simulink model "t05_balancing"  (R2024b)
settings: Solver=ode23t  StartTime=0.0  StopTime=6  RelTol=1e-3  AbsTol=1e-3  EnableMultiTasking=on
InitFcn:
  | run('Parameters_pntcld.m');
model workspace (MAT data in the model file):
  A = 0.4
  Critical_Velocity = 0.01
  Damping_Factor = 1000
  Dynamic_Friction = 0.5
  Heigth_brick : Simulink.Parameter (value not decoded)
  Heigth_ramp : Simulink.Parameter (value not decoded)
  Length_brick : Simulink.Parameter (value not decoded)
  Length_ramp : Simulink.Parameter (value not decoded)
  Length_torso : Simulink.Parameter (value not decoded)
  Lower_limbs : Simulink.Parameter (value not decoded)
  Static_Friction = 0.7
  Stiffnesscoefficient = 10000
  Transition_Region_Width = 0.02
  Upper_limbs : Simulink.Parameter (value not decoded)
  Width_brick : Simulink.Parameter (value not decoded)
  Width_ramp : Simulink.Parameter (value not decoded)
  Width_torso : Simulink.Parameter (value not decoded)
  f = 1.5
  max_Joint_change = 100
  r_foot : Simulink.Parameter (value not decoded)
  sampleTime : Simulink.Parameter (value not decoded)
  t_leg : Simulink.Parameter (value not decoded)
  theta : Simulink.Parameter (value not decoded)
  transferFunVal : Simulink.Parameter (value not decoded)
symbols that are objects in the model workspace (value not decoded): Length_torso, Lower_limbs, t_leg, transferFunVal, Upper_limbs, Width_torso
undefined symbols (not defined in the file): X, Y, Z
libraries: sm_lib x87, nesl_utility x17
(part 3 of 3)

== system t05_balancing/Front Left Leg/Upper Limb ==
  BaseUpperLimb : sm_lib/Body Elements/Brick Solid  BrickDimensions=[t_leg t_leg L]  BrickDimensionsUnits=m  ExportEntireGeometry=off  InertiaType=CalculateFromGeometry  BasedOnType=Density  Density=1000  DensityUnits=kg/m^3  Mass=1  MassUnits=kg  CenterOfMass=[0 0 0]  CenterOfMassUnits=m  MomentsOfInertia=[1 1 1]  MomentsOfInertiaUnits=kg*m^2  ProductsOfInertia=[0 0 0]  ProductsOfInertiaUnits=kg*m^2  GraphicType=FromGeometry  MarkerShape=Sphere  MarkerSize=10  GraphicVisPropType=SimpleVisualProperties  GraphicDiffuseColor=[0.502 0.502 0.502]  GraphicOpacity=1  GraphicSpecularColor=[0.5 0.5 0.5 1.0]  GraphicAmbientColor=[0.15 0.15 0.15 1.0]  GraphicEmissiveColor=[0.0 0.0 0.0 1.0]  GraphicShininess=75  DoExposeReferenceFrame=off  SerializedFrames=<Frames><Frame><Id>Frame1</Id><Value><Name>B</Name><Origin><Source>GeometricFeature</Source><FeatureName>+z surface</FeatureName></Origin><PrimaryAxis><DefinedDirection>+Z</DefinedDirection><Source>ReferenceFrame</Source><SourceDirection>+Z</SourceDirection><FeatureName></FeatureName></PrimaryAxis><SecondaryAxis><DefinedDirection>+X</DefinedDirection><Source>ReferenceFrame</Source><SourceDirection>+X</SourceDirection><FeatureName></FeatureName></SecondaryAxis></Value></Frame><Frame><Id>Frame2</Id><Value><Name>F</Name><Origin><Source>GeometricFeature</Source><FeatureName>-z surface</FeatureName></Origin><PrimaryAxis><DefinedDirection>+Z</DefinedDirection><Source>ReferenceFrame</Source><SourceDirection>+Z</SourceDirection><FeatureName></FeatureName></PrimaryAxis><SecondaryAxis><DefinedDirection>+X</DefinedDirection><Source>ReferenceFrame</Source><SourceDirection>+X</SourceDirection><FeatureName></FeatureName></SecondaryAxis></Value></Frame></Frames>
  Transform Shoulder : sm_lib/Frames and Transforms/Rigid Transform  RotationMethod=StandardAxis  FollAlignAxisA=+X  BaseAlignAxisA=+Y  FollAlignAxisB=+Y  BaseAlignAxisB=+Z  RotationStandardAxis=+X  RotationAngle=-90  RotationAngleUnits=deg  RotationArbitraryAxis=[0 0 1]  RotationSequenceAxes=FollowerAxes  RotationSequence=XYX  RotationSequenceAngles=[0 0 0]  RotationSequenceAnglesUnits=deg  RotationMatrix=[1 0 0;0 1 0;0 0 1]  Quaternion=[1 0 0 0]  TranslationMethod=StandardAxis  TranslationCartesianOffset=[0 0 0]  TranslationCartesianOffsetUnits=m  TranslationStandardAxis=+Z  TranslationStandardOffset=0  TranslationStandardOffsetUnits=m  TranslationROffset=0  TranslationROffsetUnits=m  TranslationThetaOffset=0  TranslationThetaOffsetUnits=deg  TranslationZOffset=0  TranslationZOffsetUnits=m
  Transform Upper Knee : sm_lib/Frames and Transforms/Rigid Transform  RotationMethod=StandardAxis  FollAlignAxisA=+X  BaseAlignAxisA=+Y  FollAlignAxisB=+Y  BaseAlignAxisB=+Z  RotationStandardAxis=+X  RotationAngle=-90  RotationAngleUnits=deg  RotationArbitraryAxis=[0 0 1]  RotationSequenceAxes=FollowerAxes  RotationSequence=XYX  RotationSequenceAngles=[0 0 0]  RotationSequenceAnglesUnits=deg  RotationMatrix=[1 0 0;0 1 0;0 0 1]  Quaternion=[1 0 0 0]  TranslationMethod=StandardAxis  TranslationCartesianOffset=[0 0 0]  TranslationCartesianOffsetUnits=m  TranslationStandardAxis=+Z  TranslationStandardOffset=0  TranslationStandardOffsetUnits=m  TranslationROffset=0  TranslationROffsetUnits=m  TranslationThetaOffset=0  TranslationThetaOffsetUnits=deg  TranslationZOffset=0  TranslationZOffsetUnits=m
  U : PMIOPort  Side=Left
  L : PMIOPort  Port=2  Side=Right
  connections:
  L/RConn1 -- Transform Upper Knee/RConn1
  U/RConn1 -- Transform Shoulder/RConn1
  BaseUpperLimb/LConn1 -- Transform Shoulder/LConn1
  BaseUpperLimb/RConn1 -- Transform Upper Knee/LConn1

== system t05_balancing/Front Right Leg/Lower Limb ==
  BaseLowerLimb : sm_lib/Body Elements/Brick Solid  BrickDimensions=[t_leg t_leg L]  BrickDimensionsUnits=m  ExportEntireGeometry=off  InertiaType=CalculateFromGeometry  BasedOnType=Density  Density=1000  DensityUnits=kg/m^3  Mass=1  MassUnits=kg  CenterOfMass=[0 0 0]  CenterOfMassUnits=m  MomentsOfInertia=[1 1 1]  MomentsOfInertiaUnits=kg*m^2  ProductsOfInertia=[0 0 0]  ProductsOfInertiaUnits=kg*m^2  GraphicType=FromGeometry  MarkerShape=Sphere  MarkerSize=10  GraphicVisPropType=SimpleVisualProperties  GraphicDiffuseColor=[0.5 0.5 0.5]  GraphicOpacity=1  GraphicSpecularColor=[0.5 0.5 0.5 1.0]  GraphicAmbientColor=[0.15 0.15 0.15 1.0]  GraphicEmissiveColor=[0.0 0.0 0.0 1.0]  GraphicShininess=75  DoExposeReferenceFrame=off  SerializedFrames=<Frames><Frame><Id>Frame1</Id><Value><Name>B</Name><Origin><Source>GeometricFeature</Source><FeatureName>+z surface</FeatureName></Origin><PrimaryAxis><DefinedDirection>+Z</DefinedDirection><Source>ReferenceFrame</Source><SourceDirection>+Z</SourceDirection><FeatureName></FeatureName></PrimaryAxis><SecondaryAxis><DefinedDirection>+X</DefinedDirection><Source>ReferenceFrame</Source><SourceDirection>+X</SourceDirection><FeatureName></FeatureName></SecondaryAxis></Value></Frame><Frame><Id>Frame2</Id><Value><Name>F</Name><Origin><Source>GeometricFeature</Source><FeatureName>-z surface</FeatureName></Origin><PrimaryAxis><DefinedDirection>+Z</DefinedDirection><Source>ReferenceFrame</Source><SourceDirection>+Z</SourceDirection><FeatureName></FeatureName></PrimaryAxis><SecondaryAxis><DefinedDirection>+X</DefinedDirection><Source>ReferenceFrame</Source><SourceDirection>+X</SourceDirection><FeatureName></FeatureName></SecondaryAxis></Value></Frame></Frames>
  Transform Shoulder : sm_lib/Frames and Transforms/Rigid Transform  RotationMethod=StandardAxis  FollAlignAxisA=+X  BaseAlignAxisA=+Y  FollAlignAxisB=+Y  BaseAlignAxisB=+Z  RotationStandardAxis=+X  RotationAngle=-90  RotationAngleUnits=deg  RotationArbitraryAxis=[0 0 1]  RotationSequenceAxes=FollowerAxes  RotationSequence=XYX  RotationSequenceAngles=[0 0 0]  RotationSequenceAnglesUnits=deg  RotationMatrix=[1 0 0;0 1 0;0 0 1]  Quaternion=[1 0 0 0]  TranslationMethod=StandardAxis  TranslationCartesianOffset=[0 0 0]  TranslationCartesianOffsetUnits=m  TranslationStandardAxis=+Z  TranslationStandardOffset=0  TranslationStandardOffsetUnits=m  TranslationROffset=0  TranslationROffsetUnits=m  TranslationThetaOffset=0  TranslationThetaOffsetUnits=deg  TranslationZOffset=0  TranslationZOffsetUnits=m
  Transform Upper Knee : sm_lib/Frames and Transforms/Rigid Transform  RotationMethod=StandardAxis  FollAlignAxisA=+X  BaseAlignAxisA=+Y  FollAlignAxisB=+Y  BaseAlignAxisB=+Z  RotationStandardAxis=+X  RotationAngle=-90  RotationAngleUnits=deg  RotationArbitraryAxis=[0 0 1]  RotationSequenceAxes=FollowerAxes  RotationSequence=XYX  RotationSequenceAngles=[0 0 0]  RotationSequenceAnglesUnits=deg  RotationMatrix=[1 0 0;0 1 0;0 0 1]  Quaternion=[1 0 0 0]  TranslationMethod=StandardAxis  TranslationCartesianOffset=[0 0 0]  TranslationCartesianOffsetUnits=m  TranslationStandardAxis=+Z  TranslationStandardOffset=0  TranslationStandardOffsetUnits=m  TranslationROffset=0  TranslationROffsetUnits=m  TranslationThetaOffset=0  TranslationThetaOffsetUnits=deg  TranslationZOffset=0  TranslationZOffsetUnits=m
  U : PMIOPort  Side=Left
  L : PMIOPort  Port=2  Side=Right
  connections:
  BaseLowerLimb/LConn1 -- Transform Shoulder/LConn1
  Transform Shoulder/RConn1 -- U/RConn1
  L/RConn1 -- Transform Upper Knee/RConn1
  BaseLowerLimb/RConn1 -- Transform Upper Knee/LConn1

== system t05_balancing/Front Right Leg/Upper Limb ==
  BaseUpperLimb : sm_lib/Body Elements/Brick Solid  BrickDimensions=[t_leg t_leg L]  BrickDimensionsUnits=m  ExportEntireGeometry=off  InertiaType=CalculateFromGeometry  BasedOnType=Density  Density=1000  DensityUnits=kg/m^3  Mass=1  MassUnits=kg  CenterOfMass=[0 0 0]  CenterOfMassUnits=m  MomentsOfInertia=[1 1 1]  MomentsOfInertiaUnits=kg*m^2  ProductsOfInertia=[0 0 0]  ProductsOfInertiaUnits=kg*m^2  GraphicType=FromGeometry  MarkerShape=Sphere  MarkerSize=10  GraphicVisPropType=SimpleVisualProperties  GraphicDiffuseColor=[0.502 0.502 0.502]  GraphicOpacity=1  GraphicSpecularColor=[0.5 0.5 0.5 1.0]  GraphicAmbientColor=[0.15 0.15 0.15 1.0]  GraphicEmissiveColor=[0.0 0.0 0.0 1.0]  GraphicShininess=75  DoExposeReferenceFrame=off  SerializedFrames=<Frames><Frame><Id>Frame1</Id><Value><Name>B</Name><Origin><Source>GeometricFeature</Source><FeatureName>+z surface</FeatureName></Origin><PrimaryAxis><DefinedDirection>+Z</DefinedDirection><Source>ReferenceFrame</Source><SourceDirection>+Z</SourceDirection><FeatureName></FeatureName></PrimaryAxis><SecondaryAxis><DefinedDirection>+X</DefinedDirection><Source>ReferenceFrame</Source><SourceDirection>+X</SourceDirection><FeatureName></FeatureName></SecondaryAxis></Value></Frame><Frame><Id>Frame2</Id><Value><Name>F</Name><Origin><Source>GeometricFeature</Source><FeatureName>-z surface</FeatureName></Origin><PrimaryAxis><DefinedDirection>+Z</DefinedDirection><Source>ReferenceFrame</Source><SourceDirection>+Z</SourceDirection><FeatureName></FeatureName></PrimaryAxis><SecondaryAxis><DefinedDirection>+X</DefinedDirection><Source>ReferenceFrame</Source><SourceDirection>+X</SourceDirection><FeatureName></FeatureName></SecondaryAxis></Value></Frame></Frames>
  Transform Shoulder : sm_lib/Frames and Transforms/Rigid Transform  RotationMethod=StandardAxis  FollAlignAxisA=+X  BaseAlignAxisA=+Y  FollAlignAxisB=+Y  BaseAlignAxisB=+Z  RotationStandardAxis=+X  RotationAngle=-90  RotationAngleUnits=deg  RotationArbitraryAxis=[0 0 1]  RotationSequenceAxes=FollowerAxes  RotationSequence=XYX  RotationSequenceAngles=[0 0 0]  RotationSequenceAnglesUnits=deg  RotationMatrix=[1 0 0;0 1 0;0 0 1]  Quaternion=[1 0 0 0]  TranslationMethod=StandardAxis  TranslationCartesianOffset=[0 0 0]  TranslationCartesianOffsetUnits=m  TranslationStandardAxis=+Z  TranslationStandardOffset=0  TranslationStandardOffsetUnits=m  TranslationROffset=0  TranslationROffsetUnits=m  TranslationThetaOffset=0  TranslationThetaOffsetUnits=deg  TranslationZOffset=0  TranslationZOffsetUnits=m
  Transform Upper Knee : sm_lib/Frames and Transforms/Rigid Transform  RotationMethod=StandardAxis  FollAlignAxisA=+X  BaseAlignAxisA=+Y  FollAlignAxisB=+Y  BaseAlignAxisB=+Z  RotationStandardAxis=+X  RotationAngle=-90  RotationAngleUnits=deg  RotationArbitraryAxis=[0 0 1]  RotationSequenceAxes=FollowerAxes  RotationSequence=XYX  RotationSequenceAngles=[0 0 0]  RotationSequenceAnglesUnits=deg  RotationMatrix=[1 0 0;0 1 0;0 0 1]  Quaternion=[1 0 0 0]  TranslationMethod=StandardAxis  TranslationCartesianOffset=[0 0 0]  TranslationCartesianOffsetUnits=m  TranslationStandardAxis=+Z  TranslationStandardOffset=0  TranslationStandardOffsetUnits=m  TranslationROffset=0  TranslationROffsetUnits=m  TranslationThetaOffset=0  TranslationThetaOffsetUnits=deg  TranslationZOffset=0  TranslationZOffsetUnits=m
  U : PMIOPort  Side=Left
  L : PMIOPort  Port=2  Side=Right
  connections:
  L/RConn1 -- Transform Upper Knee/RConn1
  U/RConn1 -- Transform Shoulder/RConn1
  BaseUpperLimb/LConn1 -- Transform Shoulder/LConn1
  BaseUpperLimb/RConn1 -- Transform Upper Knee/LConn1

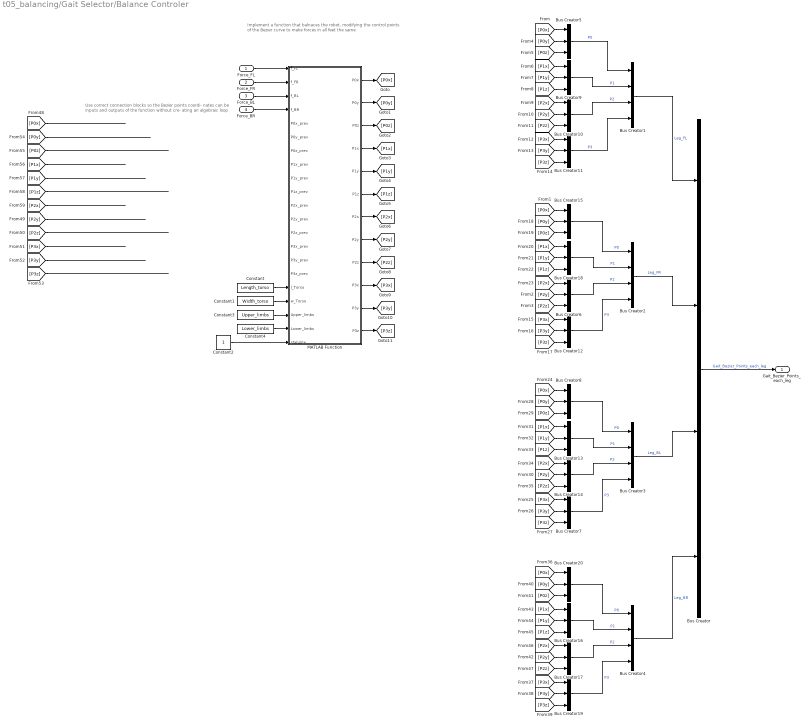
== system t05_balancing/Gait Selector/Balance Controler ==
  note: Implement a function that balnaces the robot, modifying
      | the control points of the Bezier curve to make forces in all
      | feet the same
  note: Use correct connection blocks so the Bezier points coordi-
      | nates can be inputs and outputs of the function without cre-
      | ating an algebraic loop
  Force_FL : Inport
  Force_FR : Inport  Port=2
  Force_BL : Inport  Port=3
  Force_BR : Inport  Port=4
  Bus Creator{,1..4} (5 alike) : BusCreator  Inputs=4
  Bus Creator{5..20} (16 alike) : BusCreator  Inputs=3
  Constant : Constant  Value=Length_torso
  Constant1 : Constant  Value=Width_torso
  Constant2 : Constant
  Constant3 : Constant  Value=Upper_limbs
  Constant4 : Constant  Value=Lower_limbs
  MATLAB Function : MATLAB Function  TreatAsAtomicUnit=on
  Gait_Bezier_Points_each_leg : Outport
  wires:
  Constant2/1 -> MATLAB Function/21(stabilize)
  Constant4/1 -> MATLAB Function/20(Lower_limbs)
  Constant3/1 -> MATLAB Function/19(Upper_limbs)
  ? -> MATLAB Function/13(P2z_prev)
  ? -> MATLAB Function/14(P3x_prev)
  ? -> MATLAB Function/10(P1z_prev)
  ? -> MATLAB Function/8(P1x_prev)
  ? -> MATLAB Function/12(P2y_prev)
  ? -> MATLAB Function/9(P1y_prev)
  ? -> MATLAB Function/11(P2x_prev)
  ? -> MATLAB Function/5(P0x_prev)
  ? -> MATLAB Function/15(P3y_prev)
  ? -> MATLAB Function/7(P0z_prev)
  ? -> MATLAB Function/16(P3z_prev)
  ? -> MATLAB Function/6(P0y_prev)
  [P3y] -> ?
  [P3z] -> ?
  [P3x] -> ?
  [P2x] -> ?
  [P2z] -> ?
  [P2y] -> ?
  Bus Creator20/1 -> Bus Creator4/1  "P0"
  Bus Creator16/1 -> Bus Creator4/2  "P1"
  Bus Creator17/1 -> Bus Creator4/3  "P2"
  Bus Creator19/1 -> Bus Creator4/4  "P3"
  [P0x] -> Bus Creator20/1
  [P0y] -> Bus Creator20/2
  [P0z] -> Bus Creator20/3
  [P1y] -> Bus Creator16/2
  [P1x] -> Bus Creator16/1
  [P1z] -> Bus Creator16/3
  [P3z] -> Bus Creator19/3
  [P3x] -> Bus Creator19/1
  [P3y] -> Bus Creator19/2
  [P2z] -> Bus Creator17/3
  [P2y] -> Bus Creator17/2
  [P2x] -> Bus Creator17/1
  [P2x] -> Bus Creator14/1
  [P2y] -> Bus Creator14/2
  [P2z] -> Bus Creator14/3
  [P3y] -> Bus Creator7/2
  [P3x] -> Bus Creator7/1
  [P3z] -> Bus Creator7/3
  [P1z] -> Bus Creator13/3
  [P1x] -> Bus Creator13/1
  [P1y] -> Bus Creator13/2
  [P0z] -> Bus Creator8/3
  [P0y] -> Bus Creator8/2
  [P0x] -> Bus Creator8/1
  Bus Creator7/1 -> Bus Creator3/4  "P3"
  Bus Creator14/1 -> Bus Creator3/3  "P2"
  Bus Creator13/1 -> Bus Creator3/2  "P1"
  Bus Creator8/1 -> Bus Creator3/1  "P0"
  Bus Creator15/1 -> Bus Creator2/1  "P0"
  Bus Creator18/1 -> Bus Creator2/2  "P1"
  Bus Creator6/1 -> Bus Creator2/3  "P2"
  Bus Creator12/1 -> Bus Creator2/4  "P3"
  [P0x] -> Bus Creator15/1
  [P0y] -> Bus Creator15/2
  [P0z] -> Bus Creator15/3
  [P1y] -> Bus Creator18/2
  [P1x] -> Bus Creator18/1
  [P1z] -> Bus Creator18/3
  [P3z] -> Bus Creator12/3
  [P3x] -> Bus Creator12/1
  [P3y] -> Bus Creator12/2
  [P2z] -> Bus Creator6/3
  [P2y] -> Bus Creator6/2
  [P2x] -> Bus Creator6/1
  [P2x] -> Bus Creator10/1
  [P2y] -> Bus Creator10/2
  [P2z] -> Bus Creator10/3
  [P3y] -> Bus Creator11/2
  [P3x] -> Bus Creator11/1
  [P3z] -> Bus Creator11/3
  [P1z] -> Bus Creator9/3
  [P1x] -> Bus Creator9/1
  [P1y] -> Bus Creator9/2
  MATLAB Function/7(P2x) -> [P2x]
  MATLAB Function/8(P2y) -> [P2y]
  MATLAB Function/9(P2z) -> [P2z]
  MATLAB Function/12(P3z) -> [P3z]
  MATLAB Function/11(P3y) -> [P3y]
  MATLAB Function/10(P3x) -> [P3x]
  MATLAB Function/4(P1x) -> [P1x]
  MATLAB Function/5(P1y) -> [P1y]
  MATLAB Function/6(P1z) -> [P1z]
  MATLAB Function/3(P0z) -> [P0z]
  MATLAB Function/2(P0y) -> [P0y]
  [P0z] -> Bus Creator5/3
  [P0y] -> Bus Creator5/2
  [P0x] -> Bus Creator5/1
  Constant1/1 -> MATLAB Function/18(w_Torso)
  Constant/1 -> MATLAB Function/17(l_Torso)
  [P1z] -> ?
  [P1x] -> ?
  [P1y] -> ?
  [P0y] -> ?
  [P0z] -> ?
  [P0x] -> ?
  Force_BR/1 -> MATLAB Function/4(f_BR)
  Force_BL/1 -> MATLAB Function/3(f_BL)
  Force_FR/1 -> MATLAB Function/2(f_FR)
  Force_FL/1 -> MATLAB Function/1(f_FL)
  MATLAB Function/1(P0x) -> [P0x]
  Bus Creator11/1 -> Bus Creator1/4  "P3"
  Bus Creator10/1 -> Bus Creator1/3  "P2"
  Bus Creator9/1 -> Bus Creator1/2  "P1"
  Bus Creator5/1 -> Bus Creator1/1  "P0"
  Bus Creator/1 -> Gait_Bezier_Points_each_leg/1  "Gait_Bezier_Points_each_leg"
  Bus Creator4/1 -> Bus Creator/4  "Leg_BR"
  Bus Creator3/1 -> Bus Creator/3  "Leg_BL"
  Bus Creator2/1 -> Bus Creator/2  "Leg_FR"
  Bus Creator1/1 -> Bus Creator/1  "Leg_FL"

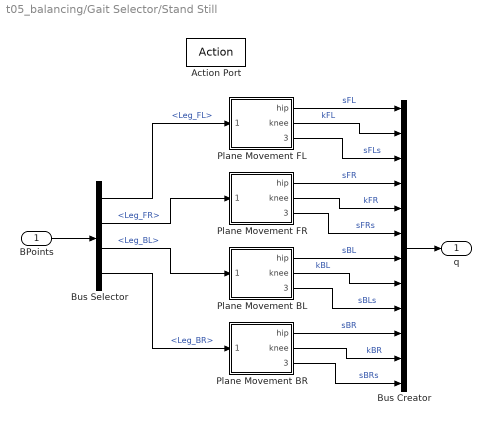
== system t05_balancing/Gait Selector/Stand Still ==
  BPoints : Inport
  Action Port : ActionPort  InitializeStates=reset  ActionPortLabel=case [ 0 ]:
  Bus Creator : BusCreator  Inputs=12
  Bus Selector : BusSelector  OutputSignals=Leg_FL,Leg_FR,Leg_BL,Leg_BR
  Plane Movement BL : Subsystem
  Plane Movement BR : Subsystem
  Plane Movement FL : Subsystem
  Plane Movement FR : Subsystem
  q : Outport
  wires:
  Bus Selector/4 -> Plane Movement BR/1(BPoints)  "<Leg_BR>"
  Bus Selector/3 -> Plane Movement BL/1(BPoints)  "<Leg_BL>"
  Bus Creator/1 -> q/1
  Plane Movement FL/1(hip) -> Bus Creator/1  "sFL"
  Plane Movement FR/1(hip) -> Bus Creator/4  "sFR"
  Plane Movement FL/2(knee) -> Bus Creator/2  "kFL"
  Plane Movement FR/2(knee) -> Bus Creator/5  "kFR"
  Plane Movement BL/2(knee) -> Bus Creator/8  "kBL"
  Plane Movement BL/1(hip) -> Bus Creator/7  "sBL"
  Plane Movement BR/2(knee) -> Bus Creator/11  "kBR"
  Plane Movement BR/1(hip) -> Bus Creator/10  "sBR"
  Plane Movement FL/3(HipLateral) -> Bus Creator/3  "sFLs"
  Plane Movement FR/3(HipLateral) -> Bus Creator/6  "sFRs"
  Plane Movement BL/3(HipLateral) -> Bus Creator/9  "sBLs"
  Plane Movement BR/3(HipLateral) -> Bus Creator/12  "sBRs"
  BPoints/1 -> Bus Selector/1
  Bus Selector/1 -> Plane Movement FL/1(BPoints)  "<Leg_FL>"
  Bus Selector/2 -> Plane Movement FR/1(BPoints)  "<Leg_FR>"

== system t05_balancing/Rear Left Leg/Lower Limb ==
  BaseLowerLimb : sm_lib/Body Elements/Brick Solid  BrickDimensions=[t_leg t_leg L]  BrickDimensionsUnits=m  ExportEntireGeometry=off  InertiaType=CalculateFromGeometry  BasedOnType=Density  Density=1000  DensityUnits=kg/m^3  Mass=1  MassUnits=kg  CenterOfMass=[0 0 0]  CenterOfMassUnits=m  MomentsOfInertia=[1 1 1]  MomentsOfInertiaUnits=kg*m^2  ProductsOfInertia=[0 0 0]  ProductsOfInertiaUnits=kg*m^2  GraphicType=FromGeometry  MarkerShape=Sphere  MarkerSize=10  GraphicVisPropType=SimpleVisualProperties  GraphicDiffuseColor=[0.5 0.5 0.5]  GraphicOpacity=1  GraphicSpecularColor=[0.5 0.5 0.5 1.0]  GraphicAmbientColor=[0.15 0.15 0.15 1.0]  GraphicEmissiveColor=[0.0 0.0 0.0 1.0]  GraphicShininess=75  DoExposeReferenceFrame=off  SerializedFrames=<Frames><Frame><Id>Frame1</Id><Value><Name>B</Name><Origin><Source>GeometricFeature</Source><FeatureName>+z surface</FeatureName></Origin><PrimaryAxis><DefinedDirection>+Z</DefinedDirection><Source>ReferenceFrame</Source><SourceDirection>+Z</SourceDirection><FeatureName></FeatureName></PrimaryAxis><SecondaryAxis><DefinedDirection>+X</DefinedDirection><Source>ReferenceFrame</Source><SourceDirection>+X</SourceDirection><FeatureName></FeatureName></SecondaryAxis></Value></Frame><Frame><Id>Frame2</Id><Value><Name>F</Name><Origin><Source>GeometricFeature</Source><FeatureName>-z surface</FeatureName></Origin><PrimaryAxis><DefinedDirection>+Z</DefinedDirection><Source>ReferenceFrame</Source><SourceDirection>+Z</SourceDirection><FeatureName></FeatureName></PrimaryAxis><SecondaryAxis><DefinedDirection>+X</DefinedDirection><Source>ReferenceFrame</Source><SourceDirection>+X</SourceDirection><FeatureName></FeatureName></SecondaryAxis></Value></Frame></Frames>
  Transform Shoulder : sm_lib/Frames and Transforms/Rigid Transform  RotationMethod=StandardAxis  FollAlignAxisA=+X  BaseAlignAxisA=+Y  FollAlignAxisB=+Y  BaseAlignAxisB=+Z  RotationStandardAxis=+X  RotationAngle=-90  RotationAngleUnits=deg  RotationArbitraryAxis=[0 0 1]  RotationSequenceAxes=FollowerAxes  RotationSequence=XYX  RotationSequenceAngles=[0 0 0]  RotationSequenceAnglesUnits=deg  RotationMatrix=[1 0 0;0 1 0;0 0 1]  Quaternion=[1 0 0 0]  TranslationMethod=StandardAxis  TranslationCartesianOffset=[0 0 0]  TranslationCartesianOffsetUnits=m  TranslationStandardAxis=+Z  TranslationStandardOffset=0  TranslationStandardOffsetUnits=m  TranslationROffset=0  TranslationROffsetUnits=m  TranslationThetaOffset=0  TranslationThetaOffsetUnits=deg  TranslationZOffset=0  TranslationZOffsetUnits=m
  Transform Upper Knee : sm_lib/Frames and Transforms/Rigid Transform  RotationMethod=StandardAxis  FollAlignAxisA=+X  BaseAlignAxisA=+Y  FollAlignAxisB=+Y  BaseAlignAxisB=+Z  RotationStandardAxis=+X  RotationAngle=-90  RotationAngleUnits=deg  RotationArbitraryAxis=[0 0 1]  RotationSequenceAxes=FollowerAxes  RotationSequence=XYX  RotationSequenceAngles=[0 0 0]  RotationSequenceAnglesUnits=deg  RotationMatrix=[1 0 0;0 1 0;0 0 1]  Quaternion=[1 0 0 0]  TranslationMethod=StandardAxis  TranslationCartesianOffset=[0 0 0]  TranslationCartesianOffsetUnits=m  TranslationStandardAxis=+Z  TranslationStandardOffset=0  TranslationStandardOffsetUnits=m  TranslationROffset=0  TranslationROffsetUnits=m  TranslationThetaOffset=0  TranslationThetaOffsetUnits=deg  TranslationZOffset=0  TranslationZOffsetUnits=m
  U : PMIOPort  Side=Left
  L : PMIOPort  Port=2  Side=Right
  connections:
  BaseLowerLimb/LConn1 -- Transform Shoulder/LConn1
  Transform Shoulder/RConn1 -- U/RConn1
  L/RConn1 -- Transform Upper Knee/RConn1
  BaseLowerLimb/RConn1 -- Transform Upper Knee/LConn1

== system t05_balancing/Rear Left Leg/Upper Limb ==
  BaseUpperLimb : sm_lib/Body Elements/Brick Solid  BrickDimensions=[t_leg t_leg L]  BrickDimensionsUnits=m  ExportEntireGeometry=off  InertiaType=CalculateFromGeometry  BasedOnType=Density  Density=1000  DensityUnits=kg/m^3  Mass=1  MassUnits=kg  CenterOfMass=[0 0 0]  CenterOfMassUnits=m  MomentsOfInertia=[1 1 1]  MomentsOfInertiaUnits=kg*m^2  ProductsOfInertia=[0 0 0]  ProductsOfInertiaUnits=kg*m^2  GraphicType=FromGeometry  MarkerShape=Sphere  MarkerSize=10  GraphicVisPropType=SimpleVisualProperties  GraphicDiffuseColor=[0.502 0.502 0.502]  GraphicOpacity=1  GraphicSpecularColor=[0.5 0.5 0.5 1.0]  GraphicAmbientColor=[0.15 0.15 0.15 1.0]  GraphicEmissiveColor=[0.0 0.0 0.0 1.0]  GraphicShininess=75  DoExposeReferenceFrame=off  SerializedFrames=<Frames><Frame><Id>Frame1</Id><Value><Name>B</Name><Origin><Source>GeometricFeature</Source><FeatureName>+z surface</FeatureName></Origin><PrimaryAxis><DefinedDirection>+Z</DefinedDirection><Source>ReferenceFrame</Source><SourceDirection>+Z</SourceDirection><FeatureName></FeatureName></PrimaryAxis><SecondaryAxis><DefinedDirection>+X</DefinedDirection><Source>ReferenceFrame</Source><SourceDirection>+X</SourceDirection><FeatureName></FeatureName></SecondaryAxis></Value></Frame><Frame><Id>Frame2</Id><Value><Name>F</Name><Origin><Source>GeometricFeature</Source><FeatureName>-z surface</FeatureName></Origin><PrimaryAxis><DefinedDirection>+Z</DefinedDirection><Source>ReferenceFrame</Source><SourceDirection>+Z</SourceDirection><FeatureName></FeatureName></PrimaryAxis><SecondaryAxis><DefinedDirection>+X</DefinedDirection><Source>ReferenceFrame</Source><SourceDirection>+X</SourceDirection><FeatureName></FeatureName></SecondaryAxis></Value></Frame></Frames>
  Transform Shoulder : sm_lib/Frames and Transforms/Rigid Transform  RotationMethod=StandardAxis  FollAlignAxisA=+X  BaseAlignAxisA=+Y  FollAlignAxisB=+Y  BaseAlignAxisB=+Z  RotationStandardAxis=+X  RotationAngle=-90  RotationAngleUnits=deg  RotationArbitraryAxis=[0 0 1]  RotationSequenceAxes=FollowerAxes  RotationSequence=XYX  RotationSequenceAngles=[0 0 0]  RotationSequenceAnglesUnits=deg  RotationMatrix=[1 0 0;0 1 0;0 0 1]  Quaternion=[1 0 0 0]  TranslationMethod=StandardAxis  TranslationCartesianOffset=[0 0 0]  TranslationCartesianOffsetUnits=m  TranslationStandardAxis=+Z  TranslationStandardOffset=0  TranslationStandardOffsetUnits=m  TranslationROffset=0  TranslationROffsetUnits=m  TranslationThetaOffset=0  TranslationThetaOffsetUnits=deg  TranslationZOffset=0  TranslationZOffsetUnits=m
  Transform Upper Knee : sm_lib/Frames and Transforms/Rigid Transform  RotationMethod=StandardAxis  FollAlignAxisA=+X  BaseAlignAxisA=+Y  FollAlignAxisB=+Y  BaseAlignAxisB=+Z  RotationStandardAxis=+X  RotationAngle=-90  RotationAngleUnits=deg  RotationArbitraryAxis=[0 0 1]  RotationSequenceAxes=FollowerAxes  RotationSequence=XYX  RotationSequenceAngles=[0 0 0]  RotationSequenceAnglesUnits=deg  RotationMatrix=[1 0 0;0 1 0;0 0 1]  Quaternion=[1 0 0 0]  TranslationMethod=StandardAxis  TranslationCartesianOffset=[0 0 0]  TranslationCartesianOffsetUnits=m  TranslationStandardAxis=+Z  TranslationStandardOffset=0  TranslationStandardOffsetUnits=m  TranslationROffset=0  TranslationROffsetUnits=m  TranslationThetaOffset=0  TranslationThetaOffsetUnits=deg  TranslationZOffset=0  TranslationZOffsetUnits=m
  U : PMIOPort  Side=Left
  L : PMIOPort  Port=2  Side=Right
  connections:
  L/RConn1 -- Transform Upper Knee/RConn1
  U/RConn1 -- Transform Shoulder/RConn1
  BaseUpperLimb/LConn1 -- Transform Shoulder/LConn1
  BaseUpperLimb/RConn1 -- Transform Upper Knee/LConn1

== system t05_balancing/Rear Right Leg/Lower Limb ==
  BaseLowerLimb : sm_lib/Body Elements/Brick Solid  BrickDimensions=[t_leg t_leg L]  BrickDimensionsUnits=m  ExportEntireGeometry=off  InertiaType=CalculateFromGeometry  BasedOnType=Density  Density=1000  DensityUnits=kg/m^3  Mass=1  MassUnits=kg  CenterOfMass=[0 0 0]  CenterOfMassUnits=m  MomentsOfInertia=[1 1 1]  MomentsOfInertiaUnits=kg*m^2  ProductsOfInertia=[0 0 0]  ProductsOfInertiaUnits=kg*m^2  GraphicType=FromGeometry  MarkerShape=Sphere  MarkerSize=10  GraphicVisPropType=SimpleVisualProperties  GraphicDiffuseColor=[0.5 0.5 0.5]  GraphicOpacity=1  GraphicSpecularColor=[0.5 0.5 0.5 1.0]  GraphicAmbientColor=[0.15 0.15 0.15 1.0]  GraphicEmissiveColor=[0.0 0.0 0.0 1.0]  GraphicShininess=75  DoExposeReferenceFrame=off  SerializedFrames=<Frames><Frame><Id>Frame1</Id><Value><Name>B</Name><Origin><Source>GeometricFeature</Source><FeatureName>+z surface</FeatureName></Origin><PrimaryAxis><DefinedDirection>+Z</DefinedDirection><Source>ReferenceFrame</Source><SourceDirection>+Z</SourceDirection><FeatureName></FeatureName></PrimaryAxis><SecondaryAxis><DefinedDirection>+X</DefinedDirection><Source>ReferenceFrame</Source><SourceDirection>+X</SourceDirection><FeatureName></FeatureName></SecondaryAxis></Value></Frame><Frame><Id>Frame2</Id><Value><Name>F</Name><Origin><Source>GeometricFeature</Source><FeatureName>-z surface</FeatureName></Origin><PrimaryAxis><DefinedDirection>+Z</DefinedDirection><Source>ReferenceFrame</Source><SourceDirection>+Z</SourceDirection><FeatureName></FeatureName></PrimaryAxis><SecondaryAxis><DefinedDirection>+X</DefinedDirection><Source>ReferenceFrame</Source><SourceDirection>+X</SourceDirection><FeatureName></FeatureName></SecondaryAxis></Value></Frame></Frames>
  Transform Shoulder : sm_lib/Frames and Transforms/Rigid Transform  RotationMethod=StandardAxis  FollAlignAxisA=+X  BaseAlignAxisA=+Y  FollAlignAxisB=+Y  BaseAlignAxisB=+Z  RotationStandardAxis=+X  RotationAngle=-90  RotationAngleUnits=deg  RotationArbitraryAxis=[0 0 1]  RotationSequenceAxes=FollowerAxes  RotationSequence=XYX  RotationSequenceAngles=[0 0 0]  RotationSequenceAnglesUnits=deg  RotationMatrix=[1 0 0;0 1 0;0 0 1]  Quaternion=[1 0 0 0]  TranslationMethod=StandardAxis  TranslationCartesianOffset=[0 0 0]  TranslationCartesianOffsetUnits=m  TranslationStandardAxis=+Z  TranslationStandardOffset=0  TranslationStandardOffsetUnits=m  TranslationROffset=0  TranslationROffsetUnits=m  TranslationThetaOffset=0  TranslationThetaOffsetUnits=deg  TranslationZOffset=0  TranslationZOffsetUnits=m
  Transform Upper Knee : sm_lib/Frames and Transforms/Rigid Transform  RotationMethod=StandardAxis  FollAlignAxisA=+X  BaseAlignAxisA=+Y  FollAlignAxisB=+Y  BaseAlignAxisB=+Z  RotationStandardAxis=+X  RotationAngle=-90  RotationAngleUnits=deg  RotationArbitraryAxis=[0 0 1]  RotationSequenceAxes=FollowerAxes  RotationSequence=XYX  RotationSequenceAngles=[0 0 0]  RotationSequenceAnglesUnits=deg  RotationMatrix=[1 0 0;0 1 0;0 0 1]  Quaternion=[1 0 0 0]  TranslationMethod=StandardAxis  TranslationCartesianOffset=[0 0 0]  TranslationCartesianOffsetUnits=m  TranslationStandardAxis=+Z  TranslationStandardOffset=0  TranslationStandardOffsetUnits=m  TranslationROffset=0  TranslationROffsetUnits=m  TranslationThetaOffset=0  TranslationThetaOffsetUnits=deg  TranslationZOffset=0  TranslationZOffsetUnits=m
  U : PMIOPort  Side=Left
  L : PMIOPort  Port=2  Side=Right
  connections:
  BaseLowerLimb/LConn1 -- Transform Shoulder/LConn1
  Transform Shoulder/RConn1 -- U/RConn1
  L/RConn1 -- Transform Upper Knee/RConn1
  BaseLowerLimb/RConn1 -- Transform Upper Knee/LConn1

== system t05_balancing/Rear Right Leg/Upper Limb ==
  BaseUpperLimb : sm_lib/Body Elements/Brick Solid  BrickDimensions=[t_leg t_leg L]  BrickDimensionsUnits=m  ExportEntireGeometry=off  InertiaType=CalculateFromGeometry  BasedOnType=Density  Density=1000  DensityUnits=kg/m^3  Mass=1  MassUnits=kg  CenterOfMass=[0 0 0]  CenterOfMassUnits=m  MomentsOfInertia=[1 1 1]  MomentsOfInertiaUnits=kg*m^2  ProductsOfInertia=[0 0 0]  ProductsOfInertiaUnits=kg*m^2  GraphicType=FromGeometry  MarkerShape=Sphere  MarkerSize=10  GraphicVisPropType=SimpleVisualProperties  GraphicDiffuseColor=[0.502 0.502 0.502]  GraphicOpacity=1  GraphicSpecularColor=[0.5 0.5 0.5 1.0]  GraphicAmbientColor=[0.15 0.15 0.15 1.0]  GraphicEmissiveColor=[0.0 0.0 0.0 1.0]  GraphicShininess=75  DoExposeReferenceFrame=off  SerializedFrames=<Frames><Frame><Id>Frame1</Id><Value><Name>B</Name><Origin><Source>GeometricFeature</Source><FeatureName>+z surface</FeatureName></Origin><PrimaryAxis><DefinedDirection>+Z</DefinedDirection><Source>ReferenceFrame</Source><SourceDirection>+Z</SourceDirection><FeatureName></FeatureName></PrimaryAxis><SecondaryAxis><DefinedDirection>+X</DefinedDirection><Source>ReferenceFrame</Source><SourceDirection>+X</SourceDirection><FeatureName></FeatureName></SecondaryAxis></Value></Frame><Frame><Id>Frame2</Id><Value><Name>F</Name><Origin><Source>GeometricFeature</Source><FeatureName>-z surface</FeatureName></Origin><PrimaryAxis><DefinedDirection>+Z</DefinedDirection><Source>ReferenceFrame</Source><SourceDirection>+Z</SourceDirection><FeatureName></FeatureName></PrimaryAxis><SecondaryAxis><DefinedDirection>+X</DefinedDirection><Source>ReferenceFrame</Source><SourceDirection>+X</SourceDirection><FeatureName></FeatureName></SecondaryAxis></Value></Frame></Frames>
  Transform Shoulder : sm_lib/Frames and Transforms/Rigid Transform  RotationMethod=StandardAxis  FollAlignAxisA=+X  BaseAlignAxisA=+Y  FollAlignAxisB=+Y  BaseAlignAxisB=+Z  RotationStandardAxis=+X  RotationAngle=-90  RotationAngleUnits=deg  RotationArbitraryAxis=[0 0 1]  RotationSequenceAxes=FollowerAxes  RotationSequence=XYX  RotationSequenceAngles=[0 0 0]  RotationSequenceAnglesUnits=deg  RotationMatrix=[1 0 0;0 1 0;0 0 1]  Quaternion=[1 0 0 0]  TranslationMethod=StandardAxis  TranslationCartesianOffset=[0 0 0]  TranslationCartesianOffsetUnits=m  TranslationStandardAxis=+Z  TranslationStandardOffset=0  TranslationStandardOffsetUnits=m  TranslationROffset=0  TranslationROffsetUnits=m  TranslationThetaOffset=0  TranslationThetaOffsetUnits=deg  TranslationZOffset=0  TranslationZOffsetUnits=m
  Transform Upper Knee : sm_lib/Frames and Transforms/Rigid Transform  RotationMethod=StandardAxis  FollAlignAxisA=+X  BaseAlignAxisA=+Y  FollAlignAxisB=+Y  BaseAlignAxisB=+Z  RotationStandardAxis=+X  RotationAngle=-90  RotationAngleUnits=deg  RotationArbitraryAxis=[0 0 1]  RotationSequenceAxes=FollowerAxes  RotationSequence=XYX  RotationSequenceAngles=[0 0 0]  RotationSequenceAnglesUnits=deg  RotationMatrix=[1 0 0;0 1 0;0 0 1]  Quaternion=[1 0 0 0]  TranslationMethod=StandardAxis  TranslationCartesianOffset=[0 0 0]  TranslationCartesianOffsetUnits=m  TranslationStandardAxis=+Z  TranslationStandardOffset=0  TranslationStandardOffsetUnits=m  TranslationROffset=0  TranslationROffsetUnits=m  TranslationThetaOffset=0  TranslationThetaOffsetUnits=deg  TranslationZOffset=0  TranslationZOffsetUnits=m
  U : PMIOPort  Side=Left
  L : PMIOPort  Port=2  Side=Right
  connections:
  L/RConn1 -- Transform Upper Knee/RConn1
  U/RConn1 -- Transform Shoulder/RConn1
  BaseUpperLimb/LConn1 -- Transform Shoulder/LConn1
  BaseUpperLimb/RConn1 -- Transform Upper Knee/LConn1

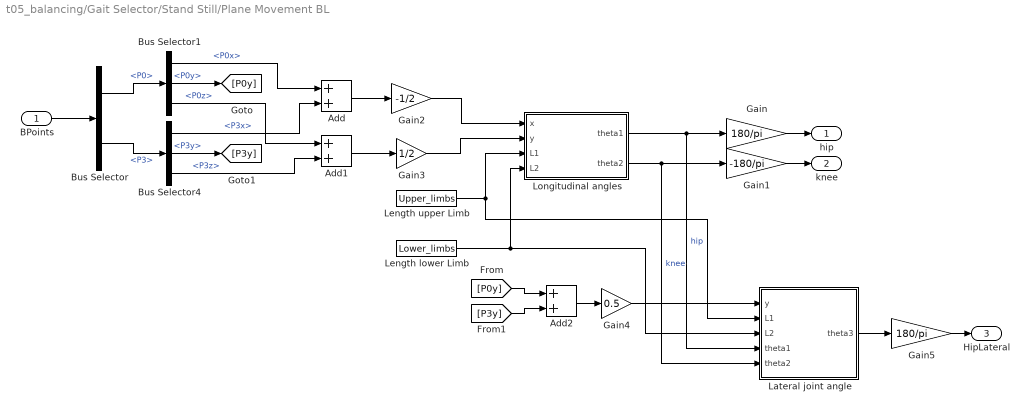
== system t05_balancing/Gait Selector/Stand Still/Plane Movement BL ==
  BPoints : Inport
  Add : Sum
  Add1 : Sum
  Add2 : Sum
  Bus Selector : BusSelector  OutputSignals=P0,P3
  Bus Selector1 : BusSelector  OutputSignals=P0x,P0y,P0z
  Bus Selector4 : BusSelector  OutputSignals=P3x,P3y,P3z
  Gain : Gain  Gain=180/pi
  Gain1 : Gain  Gain=-180/pi
  Gain2 : Gain  Gain=-1/2
  Gain3 : Gain  Gain=1/2
  Gain4 : Gain  Gain=0.5
  Gain5 : Gain  Gain=180/pi
  Lateral joint angle : MATLAB Function  TreatAsAtomicUnit=on
  Length lower Limb : Constant  Value=Lower_limbs
  Length upper Limb : Constant  Value=Upper_limbs
  Longitudinal angles : MATLAB Function  TreatAsAtomicUnit=on
  hip : Outport
  knee : Outport  Port=2
  HipLateral : Outport  Port=3
  wires:
  Gain4/1 -> Lateral joint angle/1(y)
  [P0y] -> Add2/1
  [P3y] -> Add2/2
  Gain5/1 -> HipLateral/1
  Add2/1 -> Gain4/1
  Lateral joint angle/1(theta3) -> Gain5/1
  Bus Selector4/2 -> [P3y]  "<P3y>"
  Bus Selector1/2 -> [P0y]  "<P0y>"
  BPoints/1 -> Bus Selector/1
  Gain2/1 -> Longitudinal angles/1(x)
  Add1/1 -> Gain3/1
  Add/1 -> Gain2/1
  Bus Selector4/3 -> Add1/2  "<P3z>"
  Gain3/1 -> Longitudinal angles/2(y)
  Bus Selector4/1 -> Add/2  "<P3x>"
  Gain/1 -> hip/1
  Gain1/1 -> knee/1
  Length lower Limb/1 -> Lateral joint angle/3(L2), Longitudinal angles/4(L2)
  Length upper Limb/1 -> Lateral joint angle/2(L1), Longitudinal angles/3(L1)
  Longitudinal angles/1(theta1) -> Lateral joint angle/4(theta1), Gain/1  "hip"
  Longitudinal angles/2(theta2) -> Gain1/1, Lateral joint angle/5(theta2)  "knee"
  Bus Selector/1 -> Bus Selector1/1  "<P0>"
  Bus Selector/2 -> Bus Selector4/1  "<P3>"
  Bus Selector1/1 -> Add/1  "<P0x>"
  Bus Selector1/3 -> Add1/1  "<P0z>"

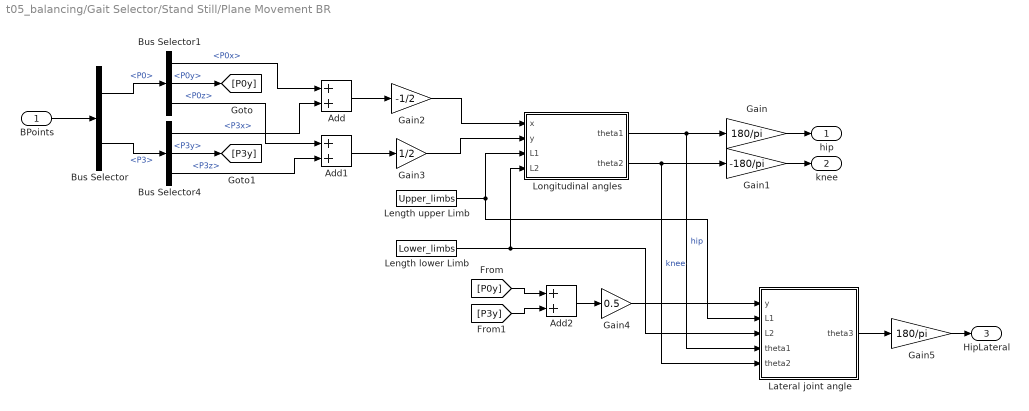
== system t05_balancing/Gait Selector/Stand Still/Plane Movement BR ==
  BPoints : Inport
  Add : Sum
  Add1 : Sum
  Add2 : Sum
  Bus Selector : BusSelector  OutputSignals=P0,P3
  Bus Selector1 : BusSelector  OutputSignals=P0x,P0y,P0z
  Bus Selector4 : BusSelector  OutputSignals=P3x,P3y,P3z
  Gain : Gain  Gain=180/pi
  Gain1 : Gain  Gain=-180/pi
  Gain2 : Gain  Gain=-1/2
  Gain3 : Gain  Gain=1/2
  Gain4 : Gain  Gain=0.5
  Gain5 : Gain  Gain=180/pi
  Lateral joint angle : MATLAB Function  TreatAsAtomicUnit=on
  Length lower Limb : Constant  Value=Lower_limbs
  Length upper Limb : Constant  Value=Upper_limbs
  Longitudinal angles : MATLAB Function  TreatAsAtomicUnit=on
  hip : Outport
  knee : Outport  Port=2
  HipLateral : Outport  Port=3
  wires:
  Gain4/1 -> Lateral joint angle/1(y)
  [P0y] -> Add2/1
  [P3y] -> Add2/2
  Gain5/1 -> HipLateral/1
  Add2/1 -> Gain4/1
  Lateral joint angle/1(theta3) -> Gain5/1
  Bus Selector4/2 -> [P3y]  "<P3y>"
  Bus Selector1/2 -> [P0y]  "<P0y>"
  BPoints/1 -> Bus Selector/1
  Gain2/1 -> Longitudinal angles/1(x)
  Add1/1 -> Gain3/1
  Add/1 -> Gain2/1
  Bus Selector4/3 -> Add1/2  "<P3z>"
  Gain3/1 -> Longitudinal angles/2(y)
  Bus Selector4/1 -> Add/2  "<P3x>"
  Gain/1 -> hip/1
  Gain1/1 -> knee/1
  Length lower Limb/1 -> Lateral joint angle/3(L2), Longitudinal angles/4(L2)
  Length upper Limb/1 -> Lateral joint angle/2(L1), Longitudinal angles/3(L1)
  Longitudinal angles/1(theta1) -> Lateral joint angle/4(theta1), Gain/1  "hip"
  Longitudinal angles/2(theta2) -> Gain1/1, Lateral joint angle/5(theta2)  "knee"
  Bus Selector/1 -> Bus Selector1/1  "<P0>"
  Bus Selector/2 -> Bus Selector4/1  "<P3>"
  Bus Selector1/1 -> Add/1  "<P0x>"
  Bus Selector1/3 -> Add1/1  "<P0z>"

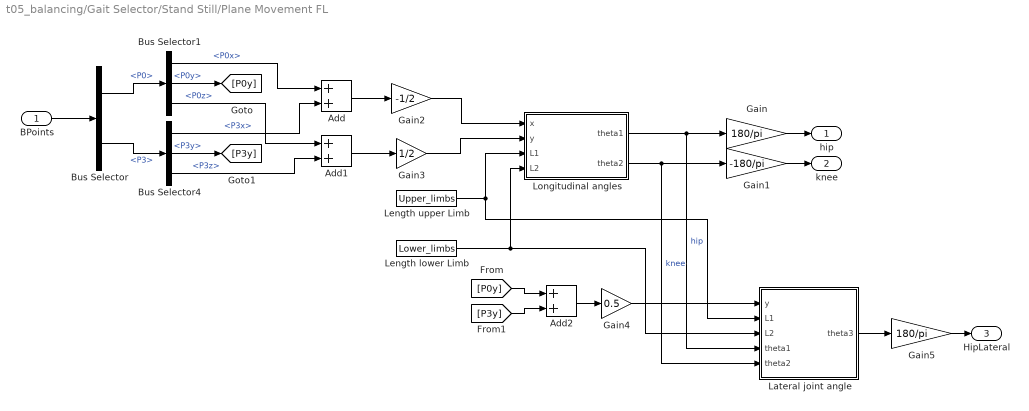
== system t05_balancing/Gait Selector/Stand Still/Plane Movement FL ==
  BPoints : Inport
  Add : Sum
  Add1 : Sum
  Add2 : Sum
  Bus Selector : BusSelector  OutputSignals=P0,P3
  Bus Selector1 : BusSelector  OutputSignals=P0x,P0y,P0z
  Bus Selector4 : BusSelector  OutputSignals=P3x,P3y,P3z
  Gain : Gain  Gain=180/pi
  Gain1 : Gain  Gain=-180/pi
  Gain2 : Gain  Gain=-1/2
  Gain3 : Gain  Gain=1/2
  Gain4 : Gain  Gain=0.5
  Gain5 : Gain  Gain=180/pi
  Lateral joint angle : MATLAB Function  TreatAsAtomicUnit=on
  Length lower Limb : Constant  Value=Lower_limbs
  Length upper Limb : Constant  Value=Upper_limbs
  Longitudinal angles : MATLAB Function  TreatAsAtomicUnit=on
  hip : Outport
  knee : Outport  Port=2
  HipLateral : Outport  Port=3
  wires:
  Gain4/1 -> Lateral joint angle/1(y)
  [P0y] -> Add2/1
  [P3y] -> Add2/2
  Gain5/1 -> HipLateral/1
  Add2/1 -> Gain4/1
  Lateral joint angle/1(theta3) -> Gain5/1
  Bus Selector4/2 -> [P3y]  "<P3y>"
  Bus Selector1/2 -> [P0y]  "<P0y>"
  BPoints/1 -> Bus Selector/1
  Gain2/1 -> Longitudinal angles/1(x)
  Add1/1 -> Gain3/1
  Add/1 -> Gain2/1
  Bus Selector4/3 -> Add1/2  "<P3z>"
  Gain3/1 -> Longitudinal angles/2(y)
  Bus Selector4/1 -> Add/2  "<P3x>"
  Gain/1 -> hip/1
  Gain1/1 -> knee/1
  Length lower Limb/1 -> Lateral joint angle/3(L2), Longitudinal angles/4(L2)
  Length upper Limb/1 -> Lateral joint angle/2(L1), Longitudinal angles/3(L1)
  Longitudinal angles/1(theta1) -> Lateral joint angle/4(theta1), Gain/1  "hip"
  Longitudinal angles/2(theta2) -> Gain1/1, Lateral joint angle/5(theta2)  "knee"
  Bus Selector/1 -> Bus Selector1/1  "<P0>"
  Bus Selector/2 -> Bus Selector4/1  "<P3>"
  Bus Selector1/1 -> Add/1  "<P0x>"
  Bus Selector1/3 -> Add1/1  "<P0z>"

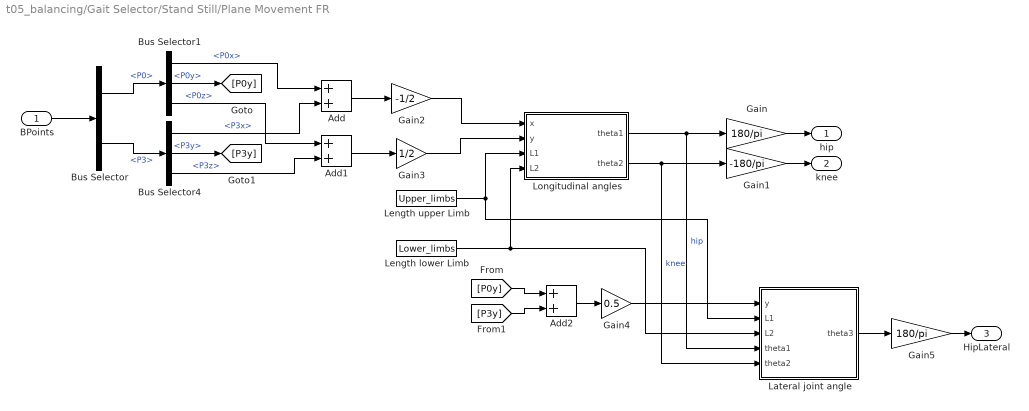
== system t05_balancing/Gait Selector/Stand Still/Plane Movement FR ==
  BPoints : Inport
  Add : Sum
  Add1 : Sum
  Add2 : Sum
  Bus Selector : BusSelector  OutputSignals=P0,P3
  Bus Selector1 : BusSelector  OutputSignals=P0x,P0y,P0z
  Bus Selector4 : BusSelector  OutputSignals=P3x,P3y,P3z
  Gain : Gain  Gain=180/pi
  Gain1 : Gain  Gain=-180/pi
  Gain2 : Gain  Gain=-1/2
  Gain3 : Gain  Gain=1/2
  Gain4 : Gain  Gain=0.5
  Gain5 : Gain  Gain=180/pi
  Lateral joint angle : MATLAB Function  TreatAsAtomicUnit=on
  Length lower Limb : Constant  Value=Lower_limbs
  Length upper Limb : Constant  Value=Upper_limbs
  Longitudinal angles : MATLAB Function  TreatAsAtomicUnit=on
  hip : Outport
  knee : Outport  Port=2
  HipLateral : Outport  Port=3
  wires:
  Gain4/1 -> Lateral joint angle/1(y)
  [P0y] -> Add2/1
  [P3y] -> Add2/2
  Gain5/1 -> HipLateral/1
  Add2/1 -> Gain4/1
  Lateral joint angle/1(theta3) -> Gain5/1
  Bus Selector4/2 -> [P3y]  "<P3y>"
  Bus Selector1/2 -> [P0y]  "<P0y>"
  BPoints/1 -> Bus Selector/1
  Gain2/1 -> Longitudinal angles/1(x)
  Add1/1 -> Gain3/1
  Add/1 -> Gain2/1
  Bus Selector4/3 -> Add1/2  "<P3z>"
  Gain3/1 -> Longitudinal angles/2(y)
  Bus Selector4/1 -> Add/2  "<P3x>"
  Gain/1 -> hip/1
  Gain1/1 -> knee/1
  Length lower Limb/1 -> Lateral joint angle/3(L2), Longitudinal angles/4(L2)
  Length upper Limb/1 -> Lateral joint angle/2(L1), Longitudinal angles/3(L1)
  Longitudinal angles/1(theta1) -> Lateral joint angle/4(theta1), Gain/1  "hip"
  Longitudinal angles/2(theta2) -> Gain1/1, Lateral joint angle/5(theta2)  "knee"
  Bus Selector/1 -> Bus Selector1/1  "<P0>"
  Bus Selector/2 -> Bus Selector4/1  "<P3>"
  Bus Selector1/1 -> Add/1  "<P0x>"
  Bus Selector1/3 -> Add1/1  "<P0z>"

== matlab function t05_balancing/Gait Selector/Stand Still/Plane Movement FR/Longitudinal angles ==
  data: x input; theta1 output; y input; L1 input; L2 input; theta2 output
function [theta1, theta2] = ang(x,y,L1,L2)
x;
y;
(x.^2+y.^2-L1.^2-L2.^2) / (2*L1*L2);
theta2 = acos((x.^2+y.^2-L1.^2-L2.^2) / (2*L1*L2));
beta = asin((L2*sin(theta2))./((x.^2+y.^2).^0.5));
theta1 = asin(x./((x.^2+y.^2).^0.5)) + beta;
end

== matlab function t05_balancing/Gait Selector/Stand Still/Plane Movement FR/Lateral joint angle ==
  data: y input; theta3 output; L1 input; L2 input; theta1 input; theta2 input
function theta3 = latAng(y, L1, L2, theta1, theta2)

l = cos(theta1)*(L1 + L2*cos(theta2));

theta3 = asin(y/l);

== matlab function t05_balancing/Gait Selector/Stand Still/Plane Movement BL/Longitudinal angles ==
  data: x input; theta1 output; y input; L1 input; L2 input; theta2 output
function [theta1, theta2] = ang(x,y,L1,L2)
x;
y;
(x.^2+y.^2-L1.^2-L2.^2) / (2*L1*L2);
theta2 = acos((x.^2+y.^2-L1.^2-L2.^2) / (2*L1*L2));
beta = asin((L2*sin(theta2))./((x.^2+y.^2).^0.5));
theta1 = asin(x./((x.^2+y.^2).^0.5)) + beta;
end

== matlab function t05_balancing/Gait Selector/Stand Still/Plane Movement BL/Lateral joint angle ==
  data: y input; theta3 output; L1 input; L2 input; theta1 input; theta2 input
function theta3 = latAng(y, L1, L2, theta1, theta2)

l = cos(theta1)*(L1 + L2*cos(theta2));

theta3 = asin(y/l);

== matlab function t05_balancing/Gait Selector/Stand Still/Plane Movement BR/Longitudinal angles ==
  data: x input; theta1 output; y input; L1 input; L2 input; theta2 output
function [theta1, theta2] = ang(x,y,L1,L2)
x;
y;
(x.^2+y.^2-L1.^2-L2.^2) / (2*L1*L2);
theta2 = acos((x.^2+y.^2-L1.^2-L2.^2) / (2*L1*L2));
beta = asin((L2*sin(theta2))./((x.^2+y.^2).^0.5));
theta1 = asin(x./((x.^2+y.^2).^0.5)) + beta;
end

== matlab function t05_balancing/Gait Selector/Stand Still/Plane Movement BR/Lateral joint angle ==
  data: y input; theta3 output; L1 input; L2 input; theta1 input; theta2 input
function theta3 = latAng(y, L1, L2, theta1, theta2)

l = cos(theta1)*(L1 + L2*cos(theta2));

theta3 = asin(y/l);

== matlab function t05_balancing/Gait Selector/Stand Still/Plane Movement FL/Longitudinal angles ==
  data: x input; theta1 output; y input; L1 input; L2 input; theta2 output
function [theta1, theta2] = ang(x,y,L1,L2)
x;
y;
(x.^2+y.^2-L1.^2-L2.^2) / (2*L1*L2);
theta2 = acos((x.^2+y.^2-L1.^2-L2.^2) / (2*L1*L2));
beta = asin((L2*sin(theta2))./((x.^2+y.^2).^0.5));
theta1 = asin(x./((x.^2+y.^2).^0.5)) + beta;
end

== matlab function t05_balancing/MATLAB Function1 ==
  data: u input; y output
function y = sumFunct(u)

y = sum(u);

== matlab function t05_balancing/MATLAB Function ==
  data: u input; y output
function y = sumFunct(u)

y = sum(u);

== matlab function t05_balancing/MATLAB Function2 ==
  data: u input; y output
function y = sumFunct(u)

y = sum(u);

== matlab function t05_balancing/MATLAB Function3 ==
  data: u input; y output
function y = sumFunct(u)

y = sum(u);

== matlab function t05_balancing/Gait Selector/Stand Still/Plane Movement FL/Lateral joint angle ==
  data: y input; theta3 output; L1 input; L2 input; theta1 input; theta2 input
function theta3 = latAng(y, L1, L2, theta1, theta2)

l = cos(theta1)*(L1 + L2*cos(theta2));

theta3 = asin(y/l);

== matlab function t05_balancing/Gait Selector/Balance Controler/MATLAB Function ==
  data: f_FL input; P0x output; P0y output; f_FR input; f_BL input; f_BR input; P0x_prev input; P0y_prev input; P0z_prev input; P1x_prev input; P1y_prev input; P1z_prev input; P2x_prev input; P2y_prev input; P2z_prev input; P3x_prev input; P3y_prev input; P3z_prev input; P0z output; P1x output; P1y output; P1z output; P2x output; P2y output; P2z output; P3x output; P3y output; P3z output; l_Torso input; w_Torso input; Upper_limbs input; Lower_limbs input; stabilize input
function [P0x,P0y,P0z,P1x,P1y,P1z,P2x,P2y,P2z,P3x,P3y,P3z] = ...
    balanceFunction(f_FL, f_FR, f_BL, f_BR,P0x_prev,P0y_prev,P0z_prev, ...
    P1x_prev,P1y_prev,P1z_prev,P2x_prev,P2y_prev,P2z_prev,P3x_prev, ...
    P3y_prev,P3z_prev,l_Torso, w_Torso, Upper_limbs, Lower_limbs, stabilize)

if abs(f_FL * f_FR * f_BL * f_BR * stabilize) < 1e-8
    P0x = P0x_prev;
    P0y = P0y_prev;
    P0z = P0z_prev;
    P1x = P1x_prev;
    P1y = P1y_prev;
    P1z = P1z_prev;
    P2x = P2x_prev;
    P2y = P2y_prev;
    P2z = P2z_prev;
    P3x = P3x_prev;
    P3y = P3y_prev;
    P3z = P3z_prev;
else
    

    % Correction x3
    if (P3x^2 + P3y^2 + P3z^2)*safetyFact >= (Lower_limbs + Upper_limbs)^2
        x_new = sign(P3x)*sqrt((Lower_limbs + Upper_limbs)^2/safetyFact - P3z^2);
        correction = x_new - P3x;
        P0x = P0x + correction;
        P1x = P1x + correction;
        P2x = P2x + correction;
        P3x = P3x + correction;
    end

    % Correction x0
    if (P0x^2 + P0y^2 + P0z^2)*safetyFact >= (Lower_limbs + Upper_limbs)^2
        x_new = sign(P0x)*sqrt((Lower_limbs + Upper_limbs)^2/safetyFact - P0z^2);
        correction = x_new - P0x;
        P0x = P0x + correction;
        P1x = P1x + correction;
        P2x = P2x + correction;
        P3x = P3x + correction;
    end

    % Correction y3
    if (P3x^2 + P3y^2 + P3z^2)*safetyFact >= (Lower_limbs + Upper_limbs)^2
        P0y = P0y_prev;
        P1y = P1y_prev;
        P2y = P2y_prev;
        P3y = P3y_prev;
    end

    % Correction y0
    if (P0x^2 + P0y^2 + P0z^2)*safetyFact >= (Lower_limbs + Upper_limbs)^2
        P0y = P0y_prev;
        P1y = P1y_prev;
        P2y = P2y_prev;
        P3y = P3y_prev;
    end
end
